simulink model "FFR_2_0"  (R2015a)
settings: Solver=ode45  StartTime=0.0  StopTime=15  RelTol=1e-3
values from neighbouring files (symbols this model uses):
  D = 0.015    [init_FFR_1_0.m]    (also in init_FFR_1_1.m; init_FFR_3area.m = [0.015 0.016 0.015]; init_FFR_3area_2.m = [0.015 0.016 0.015]; init_FFR_3area_3.m = [0.015 0.016 0.015])
  H = 0.0833    [init_FFR_1_0.m]    (also in init_FFR_1_1.m; init_FFR_3area.m = [0.1667 0.2017 0.1247] .* 0.5; init_FFR_3area_2.m = [0.1667 0.2017 0.1247] .* 0.5; init_FFR_3area_3.m = [0.1667 0.2017 0.1247] .* 0.5)
  Ki = -0.3    [init_FFR_1_0.m]    (also in init_FFR_1_1.m = -2; init_FFR_3area.m = [-0.3 -0.2 -0.4]; init_FFR_3area_2.m = [-0.3 -0.2 -0.4]; init_FFR_3area_3.m = [-0.3 -0.2 -0.4])
  R = 3    [init_FFR_1_0.m]    (also in init_FFR_1_1.m; init_FFR_3area.m = [3 2.73 2.82]; init_FFR_3area_2.m = [3 2.73 2.82]; init_FFR_3area_3.m = [3 2.73 2.82])
  T_g = 0.08    [init_FFR_1_0.m]    (also in init_FFR_1_1.m; init_FFR_3area.m = [0.08 0.06 0.07]; init_FFR_3area_2.m = [0.08 0.06 0.07]; init_FFR_3area_3.m = [0.08 0.06 0.07])
  T_t = 0.40    (= 0.4)    [init_FFR_1_0.m]    (also in init_FFR_1_1.m; init_FFR_3area.m = [0.40 0.44 0.30]; init_FFR_3area_2.m = [0.40 0.44 0.30]; init_FFR_3area_3.m = [0.40 0.44 0.30])
settings Model: Creator=tarje  LastModifiedBy=tarje

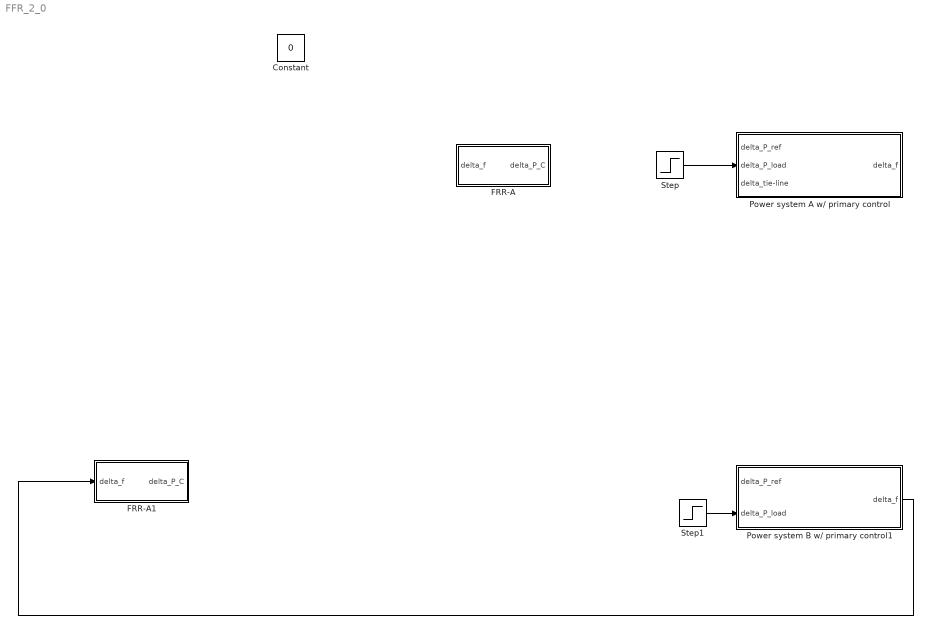
== system FFR_2_0 ==
  Constant : Constant  Value=0
  FRR-A : Subsystem
  FRR-A1 : Subsystem
  Power system A w/ primary control : Subsystem
  Power system B w/ primary control1 : Subsystem
  Step : Step  Time=2  After=.02  SampleTime=0
  Step1 : Step  Time=2  After=0  SampleTime=0
  wires:
  Step/1 -> Power system A w/ primary control/2(delta_P_load)
  Power system B w/ primary control1/1(delta_f) -> FRR-A1/1(delta_f)
  Step1/1 -> Power system B w/ primary control1/2(delta_P_load)

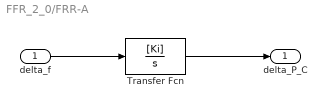
== system FFR_2_0/FRR-A ==
  delta_f : Inport
  Transfer Fcn : TransferFcn  Numerator=[Ki]  Denominator=[1 0]
  delta_P_C : Outport
  wires:
  delta_f/1 -> Transfer Fcn/1
  Transfer Fcn/1 -> delta_P_C/1

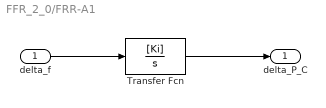
== system FFR_2_0/FRR-A1 ==
  delta_f : Inport
  Transfer Fcn : TransferFcn  Numerator=[Ki]  Denominator=[1 0]
  delta_P_C : Outport
  wires:
  delta_f/1 -> Transfer Fcn/1
  Transfer Fcn/1 -> delta_P_C/1

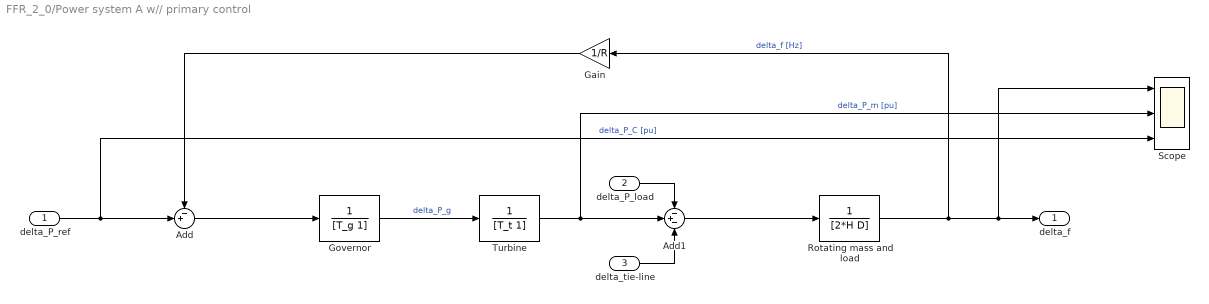
== system FFR_2_0/Power system A w// primary control ==
  delta_P_ref : Inport
  delta_P_load : Inport  Port=2
  delta_tie-line : Inport  Port=3
  Add : Sum  Inputs=-+|
  Add1 : Sum  Inputs=-+-
  Gain : Gain  Gain=1/R
  Governor : TransferFcn  Denominator=[T_g 1]
  Rotating mass and load : TransferFcn  Denominator=[2*H D]
  Scope : Scope  NumInputPorts=3
      settings: TimeRange=15  YMin=-0.08~-0.005~-0.01  YMax=0.025~0.04~0.03
  Turbine : TransferFcn  Denominator=[T_t 1]
  delta_f : Outport
  wires:
  Turbine/1 -> Add1/2, Scope/2  "delta_P_m [pu]"
  Rotating mass and load/1 -> Scope/1, delta_f/1, Gain/1  "delta_f [Hz]"
  Gain/1 -> Add/1
  Add1/1 -> Rotating mass and load/1
  Add/1 -> Governor/1
  Governor/1 -> Turbine/1  "delta_P_g"
  delta_P_ref/1 -> Scope/3, Add/2  "delta_P_C [pu]"
  delta_P_load/1 -> Add1/1
  delta_tie-line/1 -> Add1/3

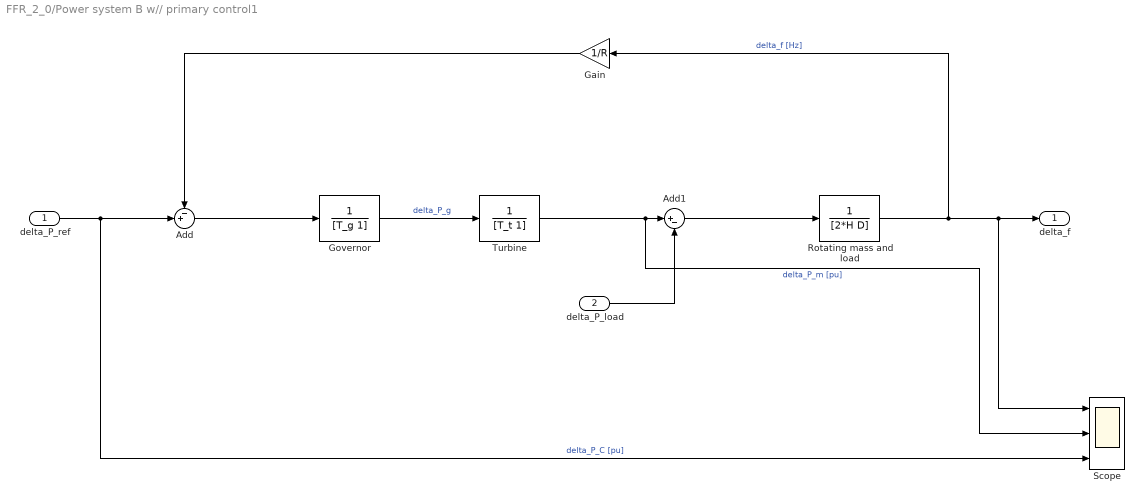
== system FFR_2_0/Power system B w// primary control1 ==
  delta_P_ref : Inport
  delta_P_load : Inport  Port=2
  Add : Sum  Inputs=-+|
  Add1 : Sum  Inputs=|+-
  Gain : Gain  Gain=1/R
  Governor : TransferFcn  Denominator=[T_g 1]
  Rotating mass and load : TransferFcn  Denominator=[2*H D]
  Scope : Scope  NumInputPorts=3
      settings: TimeRange=15  YMin=-0.08~-0.005~-0.01  YMax=0.025~0.04~0.03
  Turbine : TransferFcn  Denominator=[T_t 1]
  delta_f : Outport
  wires:
  Turbine/1 -> Scope/2, Add1/1  "delta_P_m [pu]"
  Rotating mass and load/1 -> Scope/1, delta_f/1, Gain/1  "delta_f [Hz]"
  Gain/1 -> Add/1
  delta_P_load/1 -> Add1/2
  Add1/1 -> Rotating mass and load/1
  Add/1 -> Governor/1
  Governor/1 -> Turbine/1  "delta_P_g"
  delta_P_ref/1 -> Scope/3, Add/2  "delta_P_C [pu]"
